simulink model "ISA_prob1"  (R2021a)
settings: Solver=VariableStepAuto  StartTime=0.0  StopTime=10.0  RelTol=1e-3
libraries: Atmosphere_Library x2
settings Model: Creator=prave  LastModifiedBy=prave

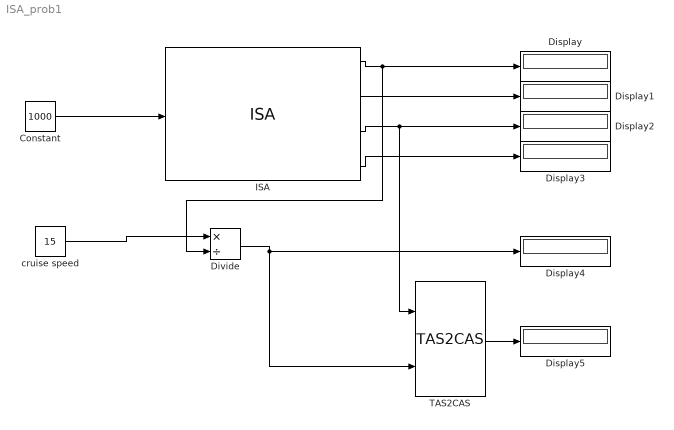
== system ISA_prob1 ==
  Constant : Constant  Value=1000
  Display{,1..5} (6 alike) : Display
  Divide : Product  Inputs=*/
  ISA : Atmosphere_Library/ISA  SystemSampleTime=-1  VariantActivationTime=update diagram  Latency=0  AutoFrameSizeCalculation=off
      link override g//(k*R): Value=-9.80665/(-0.0065*287)
  TAS2CAS : Atmosphere_Library/TAS2CAS  SystemSampleTime=-1  VariantActivationTime=update diagram  Latency=0  AutoFrameSizeCalculation=off
  cruise speed : Constant  Value=15
  wires:
  TAS2CAS/1 -> Display5/1
  ISA/2 -> Display1/1
  ISA/1 -> Display/1, Divide/2
  Divide/1 -> Display4/1, TAS2CAS/2
  ISA/3 -> Display2/1, TAS2CAS/1
  ISA/4 -> Display3/1
  Constant/1 -> ISA/1
  cruise speed/1 -> Divide/1
